simulink model "doc_scalar_quant_3"  (Simulink 5.0)
settings: Solver=ode45  StartTime=0.0  StopTime=10.0  RelTol=1e-3
undefined symbols (not defined in the file): slcm
libraries: commsrccod2 x1
settings Model: Creator=agaltman  LastModifiedBy=agaltman  ExtModeTrigMode=oneshot  ExtModeArmWhenConnect=off  LimitDataPoints=off  SignalLoggingName=logsOut  BlockReductionOpt=off  BooleanDataType=off  ZeroCrossControl=UseLocalSettings  RTWMathFcnLibMatFile=iso_c_tmw.mat

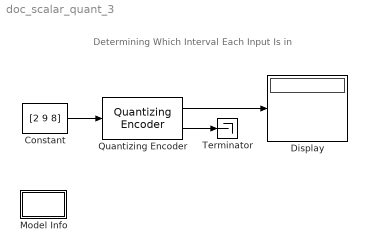
== system doc_scalar_quant_3 ==
  note: Determining Which Interval Each Input Is in
  Constant : Constant  Value=[2 9 8]
  Display : Display
  Model Info : Subsystem  LoadFcn=slcm LoadBlock;  InitFcn=slcm('UpdateAllCMBlocksInThisModelInit')  mask(CMBlock){InitialSaveTempField=, InitialBlockCM=none, BlockCM=none, Frame=on, SaveTempField=, DisplayStringWithTags=Info, MaskDisplayString=Info, HorizontalTextAlignment=Center, LeftAlignmentValue=0.5, SourceBlockDiagram=doc_scalar_quant_3, TagMaxNumber=20, CMTag1=, CMTag2=, CMTag3=, CMTag4=, CMTag5=, CMTag6=, CMTag7=, CMTag8=, CMTag9=, CMTag10=, CMTag11=, CMTag12=, CMTag13=, CMTag14=, CMTag15=, CMTag16=, CMTag17=, CMTag18=, CMTag19=, CMTag20=}
      mask help: This block allows revision control information to be displayed within the model.
      settings: CopyFcn=slcm CopyBlock;  DeleteFcn=slcm Cancel;  PostSaveFcn=slcm('UpdateAllCMBlocksInThisModel')  NameChangeFcn=slcm Rename;  OpenFcn=commdemohelp;
      mask Display: text(str2num(LeftAlignmentValue), 0.5, MaskDisplayString, 'HorizontalAlignment', HorizontalTextAlignment)
  Quantizing Encoder : commsrccod2/Quantizing Encoder  partition=[3 4 5 6 7 8 9]  codebook=ones(1,8)
  Terminator : Terminator
  wires:
  Quantizing Encoder/2 -> Terminator/1
  Constant/1 -> Quantizing Encoder/1
  Quantizing Encoder/1 -> Display/1

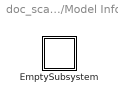
== system doc_scalar_quant_3/Model Info ==
  EmptySubsystem : Subsystem

== system doc_scalar_quant_3/Model Info/EmptySubsystem ==
